simulink model "LTV_MPC"  (R2021b)
settings: Solver=VariableStepAuto  StartTime=0.0  StopTime=15  FixedStep=0.01  RelTol=1e-3
libraries: mpclib x1
settings Model: Creator=mulusoy  LastModifiedBy=gaura
settings SolverCC: AlgebraicLoopSolver=TrustRegion
settings DataIOCC: ReturnWorkspaceOutputs=off
settings OptimizationCC: DefaultParameterBehavior=Inlined  EnhancedBackFolding=on  PassReuseOutputArgsAs=Individual arguments  OptimizeBlockOrder=speed  DifferentSizesBufferReuse=on  OptimizationCustomize=off  EfficientTunableParamExpr=on
settings DebuggingCC: ParameterTunabilityLossMsg=error  SFMachineParentedDataDiag=warning  ArithmeticOperatorsInVariantConditions=warning
settings SFSimCC: SimUseLocalCustomCode=off  MATLABDynamicMemAlloc=off  CustomCodeUndefinedFunction=UseInterfaceOnly
settings RTWCC: Description=Embedded Coder  SystemTargetFile=ert.tlc  TemplateMakefile=ert_default_tmf  GenerateReport=on  RTWUseLocalCustomCode=off  IncludeHyperlinkInReport=on  LaunchReport=on  GenerateTraceInfo=on  GenerateTraceReport=on  GenerateTraceReportSl=on  GenerateTraceReportSf=on  GenerateTraceReportEml=on
settings CodeAppCC: ForceParamTrailComments=on  IgnoreCustomStorageClasses=off  OperatorAnnotations=on  SimulinkDataObjDesc=on  SFDataObjDesc=on  InsertBlockDesc=on
settings ERTTargetCC: TargetLangStandard=C99 (ISO)  GenerateSampleERTMain=on  InlinedParameterPlacement=NonHierarchical  ERTCustomFileTemplate=example_file_process.tlc

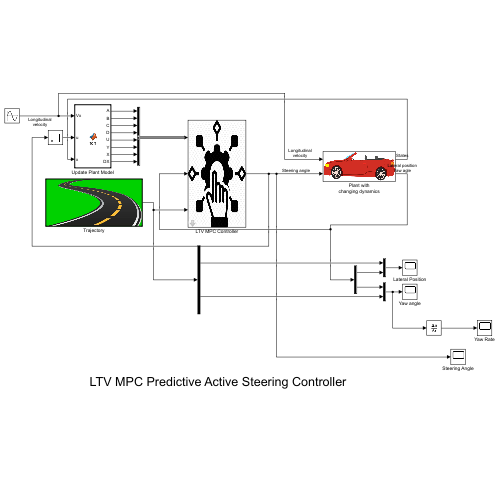
[thumbnail: Simulink's stored preview of the top-level diagram]
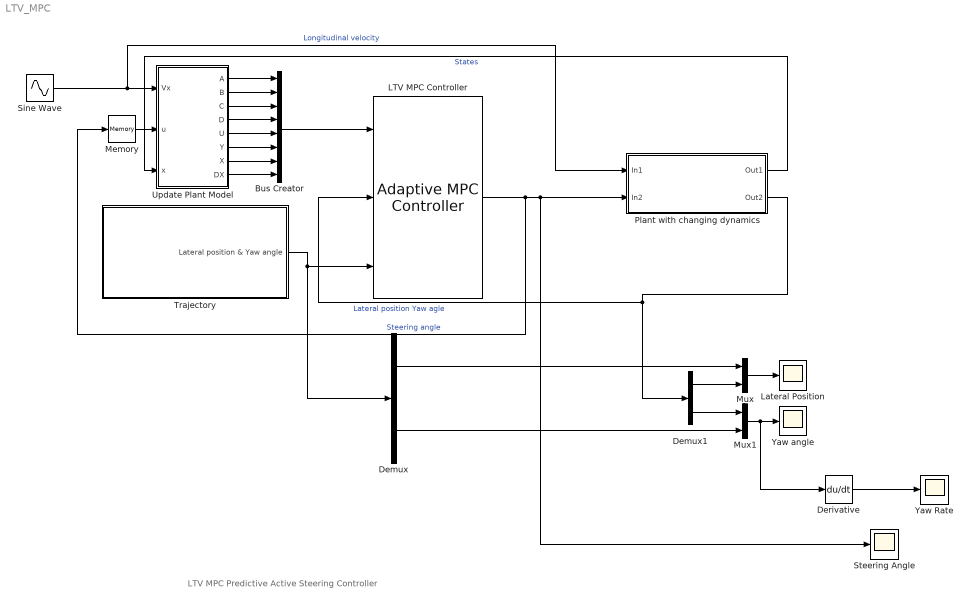
== system LTV_MPC ==
  note: LTV MPC Predictive Active Steering Controller
  Bus Creator : BusCreator  Inputs=8
  Demux : Demux  Outputs=2
  Demux1 : Demux  Outputs=2
  Derivative : Derivative
  LTV MPC Controller : mpclib/Adaptive MPC Controller  SCDEnableBlockLinearizationSpecification=on  mpcobj=mpc1  enable_value=0  updateMPCinCallerWorkspace=on  md_inport=off  mv_inport=off  uref_inport=off  return_cost=off  return_mvseq=off  return_qpstatus=off  return_xseq=off  return_state=off  return_ovseq=off  state_inport=off  isltv_plant=off  umin_inport=off  umax_inport=off  ymin_inport=off  ymax_inport=off  cc_inport=off  ywt_inport=off  uwt_inport=off  duwt_inport=off  rhoeps_inport=off  pm_inport=off  MaximumP=10  HorizonChoice=FixedHorizon  BlockDataType=double  SampleTimeInherited=off  switch_inport=off  mask(Adaptive MPC){}
      mask Display: image('LTV.png'); % Use "Edit Image" on toolstrip to change.
  Lateral Position : Scope
  Memory : Memory
  Mux : Mux  Inputs=2
  Mux1 : Mux  Inputs=2
  Plant with changing dynamics : Subsystem
      mask Display: image('convertible-car-png.png'); % Use "Edit Image" on toolstrip to change.
  Sine Wave : Sin  Amplitude=3  Bias=7  Frequency=5  SampleTime=0
  Steering Angle : Scope
  Trajectory : Subsystem  TreatAsAtomicUnit=on
      mask Display: image('road_PNG48.png'); % Use "Edit Image" on toolstrip to change.
  Update Plant Model : MATLAB Function  TreatAsAtomicUnit=on
  Yaw Rate : Scope
  Yaw angle : Scope
  wires:
  Sine Wave/1 -> Plant with changing dynamics/1(In1), Update Plant Model/1(Vx)  "Longitudinal velocity"
  Update Plant Model/1(A) -> Bus Creator/1
  Update Plant Model/2(B) -> Bus Creator/2
  Update Plant Model/3(C) -> Bus Creator/3
  Update Plant Model/4(D) -> Bus Creator/4
  Update Plant Model/5(U) -> Bus Creator/5
  Update Plant Model/6(Y) -> Bus Creator/6
  Update Plant Model/7(X) -> Bus Creator/7
  Update Plant Model/8(DX) -> Bus Creator/8
  Bus Creator/1 -> LTV MPC Controller/1
  LTV MPC Controller/1 -> Memory/1, Steering Angle/1, Plant with changing dynamics/2(In2)  "Steering angle"
  Trajectory/1(Lateral position & Yaw angle) -> LTV MPC Controller/3, Demux/1
  Demux/1 -> Mux/1
  Mux/1 -> Lateral Position/1
  Demux1/1 -> Mux/2
  Demux1/2 -> Mux1/1
  Demux/2 -> Mux1/2
  Mux1/1 -> Derivative/1, Yaw angle/1
  Plant with changing dynamics/2(Out2) -> Demux1/1, LTV MPC Controller/2  "Lateral position Yaw agle"
  Plant with changing dynamics/1(Out1) -> Update Plant Model/3(x)  "States"
  Memory/1 -> Update Plant Model/2(u)
  Derivative/1 -> Yaw Rate/1

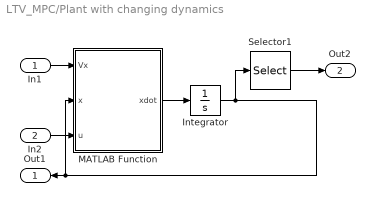
== system LTV_MPC/Plant with changing dynamics ==
  In1 : Inport
  In2 : Inport  Port=2
  Integrator : Integrator
  MATLAB Function : MATLAB Function  TreatAsAtomicUnit=on
  Selector1 : Selector  InputPortWidth=4  IndexOptions=Index vector (dialog)  Indices=[4 2]  OutputSizes=1
  Out1 : Outport  VectorParamsAs1DForOutWhenUnconnected=off
  Out2 : Outport  Port=2  VectorParamsAs1DForOutWhenUnconnected=off
  wires:
  In2/1 -> MATLAB Function/3(u)
  In1/1 -> MATLAB Function/1(Vx)
  Integrator/1 -> Selector1/1, MATLAB Function/2(x), Out1/1
  MATLAB Function/1(xdot) -> Integrator/1
  Selector1/1 -> Out2/1

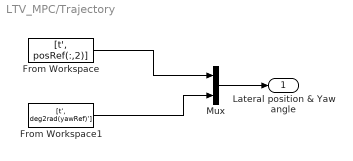
== system LTV_MPC/Trajectory ==
  From Workspace : FromWorkspace  VariableName=[t', posRef(:,2)]  SampleTime=0.1
  From Workspace1 : FromWorkspace  VariableName=[t', deg2rad(yawRef)']  SampleTime=0.1
  Mux : Mux  Inputs=2
  Lateral position & Yaw angle : Outport  VectorParamsAs1DForOutWhenUnconnected=off
  wires:
  Mux/1 -> Lateral position & Yaw angle/1
  From Workspace1/1 -> Mux/2
  From Workspace/1 -> Mux/1

== matlab function LTV_MPC/Plant with changing dynamics/MATLAB Function ==
  data: Vx input; x input size=[4,1]; u input; xdot output size=[4,1]
function xdot= fcn(Vx,x,u)

% Model parameters
m = 2050;
Iz = 3344;
lf = 1.2;
lr = 1.6;
Cf = 19000;
Cr = 33000;

% Continuous-time model
A = [-(2*Cf+2*Cr)/m/Vx, 0, -Vx-(2*Cf*lf-2*Cr*lr)/m/Vx, 0;
     0, 0, 1, 0;
     -(2*Cf*lf-2*Cr*lr)/Iz/Vx, 0, -(2*Cf*lf^2+2*Cr*lr^2)/Iz/Vx, 0;
     1, Vx, 0, 0];
B = [2*Cf/m 0 2*Cf*lf/Iz 0]';   
C = [0 0 0 1; 0 1 0 0];
D = zeros(2,1);
xdot = A*x + B*u;
y = C*x + D*u;

== matlab function LTV_MPC/Update Plant Model ==
  data: Vx input; u input; A output size=[4,4]; x input size=[4,1]; B output size=[4,1]; C output size=[2,4]; D output size=[2,1]; U output; Y output size=[2,1]; X output size=[4,1]; DX output size=[4,1]
function [A,B,C,D,U,Y,X,DX] = fcn(Vx,u,x)
% Sample time
Ts = 0.05;

% Model parameters
m = 2050;
Iz = 3344;
lf = 1.2;
lr = 1.6;
Cf = 19000;
Cr = 33000;

% Continuous-time model
Ac = [-(2*Cf+2*Cr)/m/Vx, 0, -Vx-(2*Cf*lf-2*Cr*lr)/m/Vx, 0;
     0, 0, 1, 0;
     -(2*Cf*lf-2*Cr*lr)/Iz/Vx, 0, -(2*Cf*lf^2+2*Cr*lr^2)/Iz/Vx, 0;
     1, Vx, 0, 0];
Bc = [2*Cf/m 0 2*Cf*lf/Iz 0]';   
Cc = [0 0 0 1; 0 1 0 0];
Dc = zeros(2,1);

% Generate discrete-time model
nx = size(Ac,1);
nu = size(Bc,2);
M = expm([[Ac Bc]*Ts; zeros(nu,nx+nu)]);
A = M(1:nx,1:nx);
B = M(1:nx,nx+1:nx+nu);
C = Cc;
D = Dc;

% Nominal conditions for discrete-time plant
X = x;
U = u;
Y = C*x + D*u;
DX = A*x+B*u-x;
